simulink model "controller_AWBT_2"  (R2015a)
settings: Solver=ode5  StartTime=0.0  StopTime=9  FixedStep=1e-4  RelTol=1e-3
values from neighbouring files (symbols this model uses):
  Ap = A    [main_matlab.m]    (also in plant.mat = [-1002.24784496 -454.506565622 -160.227880959 210.890100603 )
  Bp = B    [main_matlab.m]    (also in plant.mat = [-35021.5129186  -146242.93016; -63281.3491252  -264885.2852)
  Cp = C    [main_matlab.m]    (also in plant.mat = [-41.6645962626  25.6343165045  -1.45941940942  24.623653665)
  Hp = E    [main_matlab.m]    (also in plant.mat = [2997.32485293 5416.6348645 -1433.33551308 82.561739205])
  Lambda = [22.1836214239  117.354818531; -20.8929241001  -52.7332714848; 3.18075539676  -43.3165953258; 9.79046253053  -8.11991695536; -0.958677921784  -0.0562930588037; -0.0308816098304  -0.886378957674]    [controller_khat.mat]    (also in second_phase.m = X/M; second_phase_revised.m = X/M)
libraries: cstblocks x2, simulink x1
settings Model: Creator=p4wp4w  LastModifiedBy=p4wp4w
settings SolverCC: AlgebraicLoopSolver=LineSearch

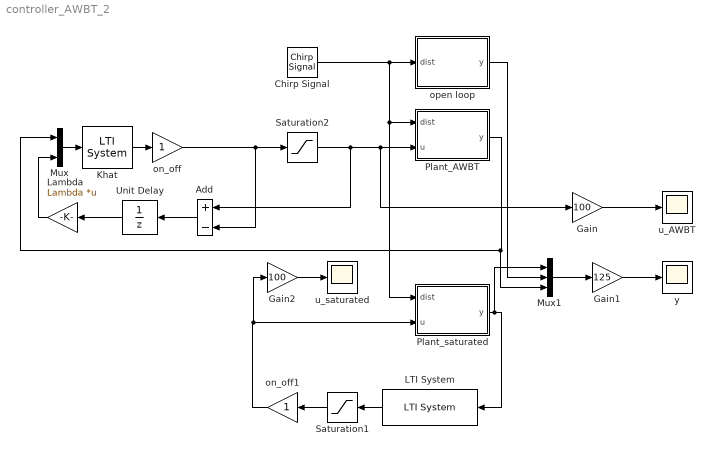
== system controller_AWBT_2 ==
  Add : Sum  Inputs=+-
  Chirp Signal : simulink/Sources/Chirp Signal  f1=0.1  T=9  f2=90
  Gain : Gain  Gain=100
  Gain1 : Gain  Gain=125
  Gain2 : Gain  Gain=100
  Khat : cstblocks/LTI System  sys=Khat  IC=[]
  LTI System : cstblocks/LTI System  sys=controller_implemented  IC=[]
  Lambda : Gain  Gain=Lambda  Multiplication=Matrix(K*u)
  Mux : Mux  Inputs=2
  Mux1 : Mux  Inputs=3
  Plant_AWBT : Subsystem
  Plant_saturated : Subsystem
  Saturation1 : Saturate  UpperLimit=2  LowerLimit=-2
  Saturation2 : Saturate  UpperLimit=2  LowerLimit=-2
  Unit Delay : UnitDelay  SampleTime=-1
  on_off : Gain
  on_off1 : Gain
  open loop : Subsystem
  u_AWBT : Scope
      settings: YMin=-0.75  YMax=0.75
  u_saturated : Scope
      settings: SaveName=ScopeData2
  y : Scope
      settings: ShowLegends=on  YMin=-4  YMax=4
  wires:
  Mux/1 -> Khat/1
  Plant_AWBT/1(y) -> Mux1/3, Mux/1
  Khat/1 -> on_off/1
  Chirp Signal/1 -> open loop/1(dist), Plant_saturated/1(dist), Plant_AWBT/1(dist)
  LTI System/1 -> Saturation1/1
  Plant_saturated/1(y) -> LTI System/1, Mux1/1
  Saturation1/1 -> on_off1/1
  Mux1/1 -> Gain1/1
  open loop/1(y) -> Mux1/2
  on_off1/1 -> Gain2/1, Plant_saturated/2(u)
  Lambda/1 -> Mux/2
  on_off/1 -> Add/2, Saturation2/1
  Saturation2/1 -> Add/1, Gain/1, Plant_AWBT/2(u)
  Add/1 -> Unit Delay/1
  Gain/1 -> u_AWBT/1
  Gain1/1 -> y/1
  Gain2/1 -> u_saturated/1
  Unit Delay/1 -> Lambda/1

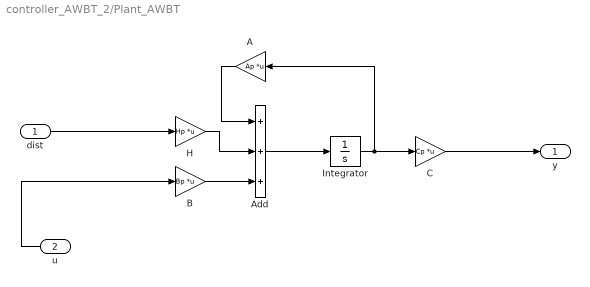
== system controller_AWBT_2/Plant_AWBT ==
  dist : Inport
  u : Inport  Port=2
  A : Gain  Gain=Ap  Multiplication=Matrix(K*u)
  Add : Sum  Inputs=+++
  B : Gain  Gain=Bp  Multiplication=Matrix(K*u)
  C : Gain  Gain=Cp  Multiplication=Matrix(K*u)
  H : Gain  Gain=Hp  Multiplication=Matrix(K*u)
  Integrator : Integrator
  y : Outport
  wires:
  Add/1 -> Integrator/1
  H/1 -> Add/2
  A/1 -> Add/1
  dist/1 -> H/1
  B/1 -> Add/3
  Integrator/1 -> C/1, A/1
  u/1 -> B/1
  C/1 -> y/1

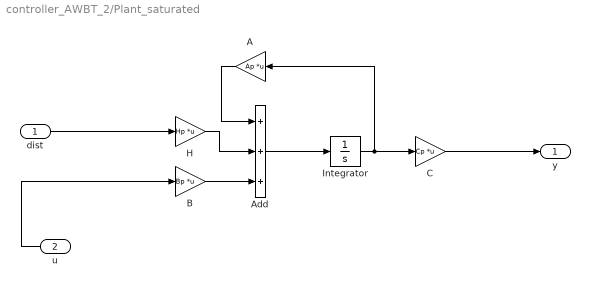
== system controller_AWBT_2/Plant_saturated ==
  dist : Inport
  u : Inport  Port=2
  A : Gain  Gain=Ap  Multiplication=Matrix(K*u)
  Add : Sum  Inputs=+++
  B : Gain  Gain=Bp  Multiplication=Matrix(K*u)
  C : Gain  Gain=Cp  Multiplication=Matrix(K*u)
  H : Gain  Gain=Hp  Multiplication=Matrix(K*u)
  Integrator : Integrator
  y : Outport
  wires:
  u/1 -> B/1
  Integrator/1 -> A/1, C/1
  B/1 -> Add/3
  dist/1 -> H/1
  A/1 -> Add/1
  H/1 -> Add/2
  Add/1 -> Integrator/1
  C/1 -> y/1

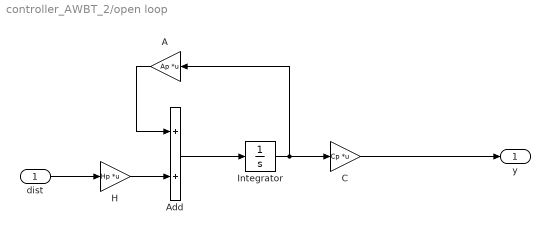
== system controller_AWBT_2/open loop ==
  dist : Inport
  A : Gain  Gain=Ap  Multiplication=Matrix(K*u)
  Add : Sum
  C : Gain  Gain=Cp  Multiplication=Matrix(K*u)
  H : Gain  Gain=Hp  Multiplication=Matrix(K*u)
  Integrator : Integrator
  y : Outport
  wires:
  Integrator/1 -> A/1, C/1
  dist/1 -> H/1
  A/1 -> Add/1
  H/1 -> Add/2
  Add/1 -> Integrator/1
  C/1 -> y/1
